simulink model "sampleModel116"  (R2021b)
settings: Solver=VariableStepAuto  StartTime=0.0  StopTime=10.0  RelTol=1e-3
undefined symbols (not defined in the file or in its folder): Newton, Raphson
libraries: simulink x5
settings Model: Creator=user  LastModifiedBy=user

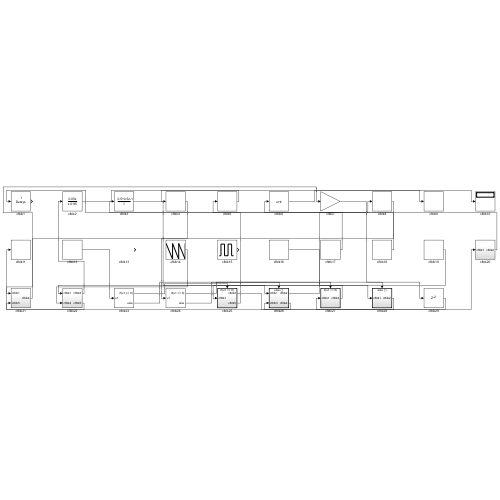
[thumbnail: Simulink's stored preview of the top-level diagram]
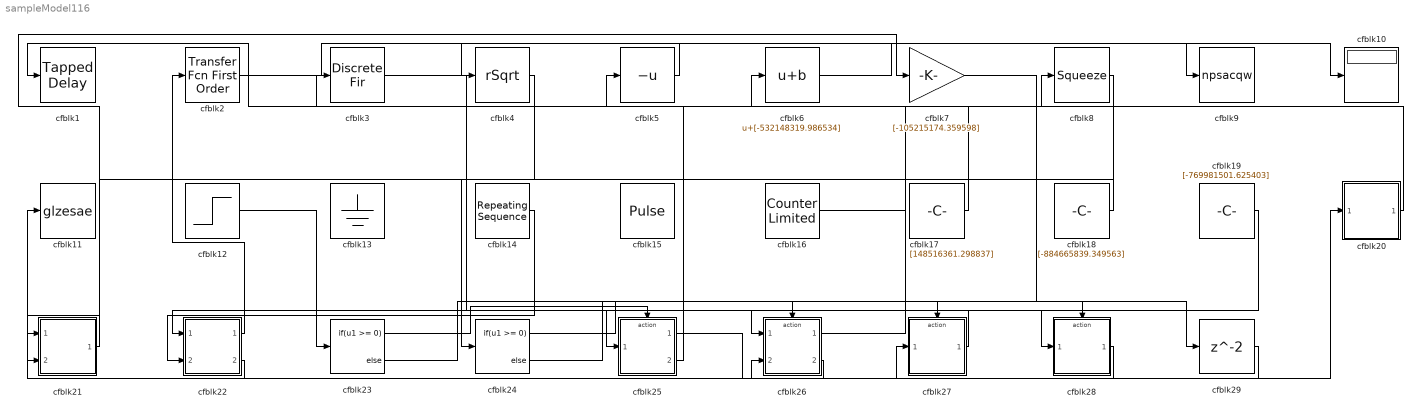
== system sampleModel116 ==
  cfblk1 : simulink/Discrete/Tapped Delay  vinit=0.0  samptime=-1  NumDelays=1  DelayOrder=Oldest  includeCurrent=off
  cfblk10 : Display
  cfblk11 : ToWorkspace  VariableName=glzesae  SaveFormat=Timeseries  SampleTime=-1
  cfblk12 : Step  Time=[33.000000]  Before=[215133831.393831]  After=[318317455.856129]  SampleTime=0
  cfblk13 : Ground
  cfblk14 : simulink/Sources/Repeating Sequence  rep_seq_t=[0 2]  rep_seq_y=[-100649541.406744, -605603657.301222]
  cfblk15 : DiscretePulseGenerator  PulseType=Time based  Amplitude=[-585443702.440842]  Period=[34836568.845558]  PulseWidth=5  PhaseDelay=[7.000000]
  cfblk16 : simulink/Sources/Counter Limited  uplimit=[101.000000]  tsamp=-1
  cfblk17 : Constant  Value=[148516361.298837]  SampleTime=1
  cfblk18 : Constant  Value=[-884665839.349563]  SampleTime=1
  cfblk19 : Constant  Value=[-769981501.625403]  SampleTime=1
  cfblk2 : simulink/Discrete/Transfer Fcn First Order  PoleZ=0.95  ICPrevOutput=0.0  DoSatur=off
  cfblk20 : Subsystem
  cfblk21 : Subsystem
  cfblk22 : Subsystem
  cfblk23 : If  IfExpression=u1 >= 0  SampleTime=1
  cfblk24 : If  IfExpression=u1 >= 0  SampleTime=1
  cfblk25 : Subsystem  TreatAsAtomicUnit=on
  cfblk26 : Subsystem  TreatAsAtomicUnit=on
  cfblk27 : Subsystem  TreatAsAtomicUnit=on
  cfblk28 : Subsystem  TreatAsAtomicUnit=on
  cfblk29 : Delay  SampleTime=1
  cfblk3 : DiscreteFir  SampleTime=1
  cfblk4 : Sqrt  Operator=rSqrt  AlgorithmType=Newton-Raphson  SaturateOnIntegerOverflow=on
  cfblk5 : UnaryMinus
  cfblk6 : Bias  Bias=[-532148319.986534]
  cfblk7 : Gain  Gain=[-105215174.359598]
  cfblk8 : Squeeze
  cfblk9 : ToWorkspace  VariableName=npsacqw  SaveFormat=Timeseries  SampleTime=-1
  wires:
  cfblk22/1(cfblk2) -> cfblk2/1
  cfblk22/2(cfblk5) -> cfblk11/1
  cfblk18/1 -> cfblk1/1
  cfblk26/1(cfblk2) -> cfblk8/1
  cfblk3/1 -> cfblk26/1(cfblk1)
  cfblk21/1(cfblk2) -> cfblk7/1
  cfblk25/1(cfblk2) -> cfblk20/1(cfblk1)
  cfblk28/1(cfblk2) -> cfblk27/1(cfblk1)
  cfblk4/1 -> cfblk24/1
  cfblk8/1 -> cfblk21/1(cfblk1)
  cfblk19/1 -> cfblk25/1(cfblk1)
  cfblk27/1(cfblk2) -> cfblk22/1(cfblk1)
  cfblk2/1 -> cfblk10/1
  cfblk26/2(cfblk4) -> cfblk21/2(cfblk5)
  cfblk16/1 -> cfblk28/1(cfblk1)
  cfblk14/1 -> cfblk22/2(cfblk4)
  cfblk17/1 -> cfblk3/1
  cfblk6/1 -> cfblk9/1
  cfblk25/2(cfblk5) -> cfblk5/1
  cfblk20/1(cfblk2) -> cfblk6/1
  cfblk5/1 -> cfblk4/1
  cfblk12/1 -> cfblk23/1
  cfblk23/1 -> cfblk25/Action
  cfblk23/2 -> cfblk26/Action
  cfblk24/1 -> cfblk27/Action
  cfblk24/2 -> cfblk28/Action
  cfblk7/1 -> cfblk29/1
  cfblk29/1 -> cfblk26/2(cfblk3)

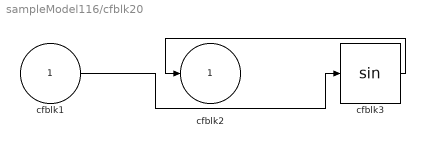
== system sampleModel116/cfblk20 ==
  cfblk1 : Inport
  cfblk3 : Trigonometry
  cfblk2 : Outport
  wires:
  cfblk3/1 -> cfblk2/1
  cfblk1/1 -> cfblk3/1

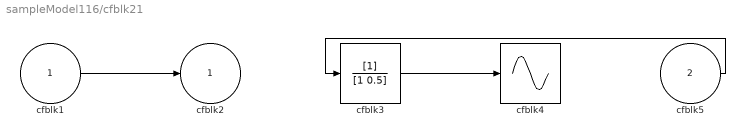
== system sampleModel116/cfblk21 ==
  cfblk1 : Inport
  cfblk5 : Inport  Port=2
  cfblk3 : DiscreteFilter  SampleTime=1
  cfblk4 : Sin  TimeSource=Use external signal  SampleTime=0
  cfblk2 : Outport
  wires:
  cfblk5/1 -> cfblk3/1
  cfblk1/1 -> cfblk2/1
  cfblk3/1 -> cfblk4/1

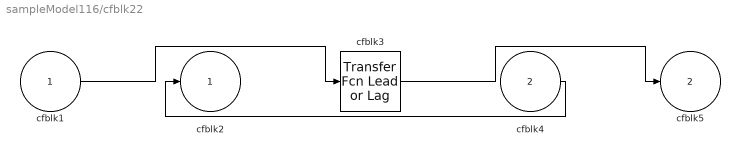
== system sampleModel116/cfblk22 ==
  cfblk1 : Inport
  cfblk4 : Inport  Port=2
  cfblk3 : simulink/Discrete/Transfer Fcn Lead or Lag  PoleZ=0.95  ZeroZ=0.75  ICPrevOutput=0.0  ICPrevInput=0.0  DoSatur=off
      settings: SourceProductBaseCode=SL
  cfblk2 : Outport
  cfblk5 : Outport  Port=2
  wires:
  cfblk3/1 -> cfblk5/1
  cfblk4/1 -> cfblk2/1
  cfblk1/1 -> cfblk3/1

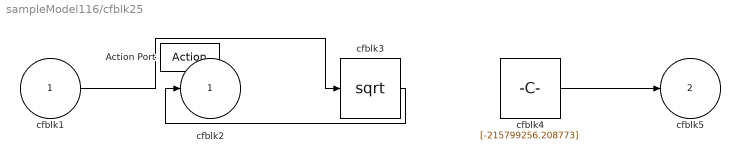
== system sampleModel116/cfblk25 ==
  cfblk1 : Inport
  Action Port : ActionPort  ActionPortLabel=if(u1 >= 0)
  cfblk3 : Sqrt  SaturateOnIntegerOverflow=on
  cfblk4 : Constant  Value=[-215799256.208773]  SampleTime=1
  cfblk2 : Outport
  cfblk5 : Outport  Port=2
  wires:
  cfblk3/1 -> cfblk2/1
  cfblk4/1 -> cfblk5/1
  cfblk1/1 -> cfblk3/1

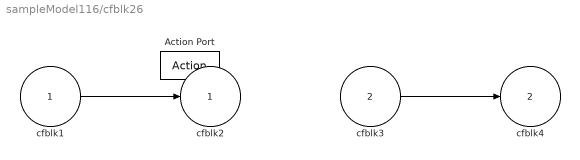
== system sampleModel116/cfblk26 ==
  cfblk1 : Inport
  cfblk3 : Inport  Port=2
  Action Port : ActionPort  ActionPortLabel=else
  cfblk2 : Outport
  cfblk4 : Outport  Port=2
  wires:
  cfblk1/1 -> cfblk2/1
  cfblk3/1 -> cfblk4/1

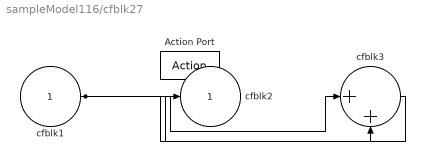
== system sampleModel116/cfblk27 ==
  cfblk1 : Inport
  Action Port : ActionPort  ActionPortLabel=if(u1 >= 0)
  cfblk3 : Sum  Inputs=|++
  cfblk2 : Outport
  wires:
  cfblk1/1 -> cfblk3/1, cfblk3/2
  cfblk3/1 -> cfblk2/1

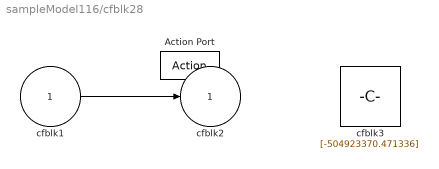
== system sampleModel116/cfblk28 ==
  cfblk1 : Inport
  Action Port : ActionPort  ActionPortLabel=else
  cfblk3 : Constant  Value=[-504923370.471336]  SampleTime=1
  cfblk2 : Outport
  wires:
  cfblk1/1 -> cfblk2/1
